simulink model "singleMassMPCDemodiscrete2017"  (R2017a)
settings: Solver=ode4  StartTime=0.0  StopTime=8  FixedStep=0.1  RelTol=1e-3
libraries: simulink x1
settings Model: Creator=daoist  LastModifiedBy=daoist
settings DataIOCC: ReturnWorkspaceOutputs=on
settings DebuggingCC: SFMachineParentedDataDiag=error
settings SFSimCC: SimUseLocalCustomCode=on
settings RTWCC: RTWUseLocalCustomCode=on

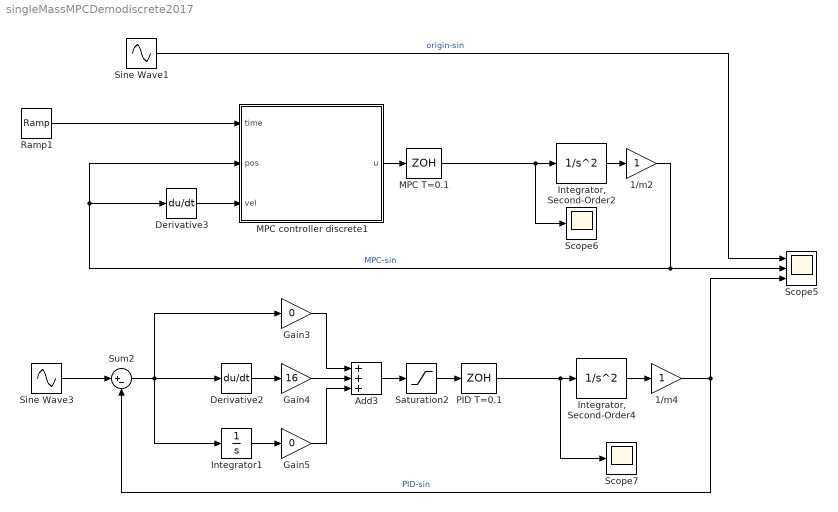
== system singleMassMPCDemodiscrete2017 ==
  1/m2 : Gain
  1/m4 : Gain
  Add3 : Sum  Inputs=+++
  Derivative2 : Derivative
  Derivative3 : Derivative
  Gain3 : Gain  Gain=0
  Gain4 : Gain  Gain=16
  Gain5 : Gain  Gain=0
  "Integrator, Second-Order2" : SecondOrderIntegrator  ShowOutput=x
  "Integrator, Second-Order4" : SecondOrderIntegrator  ShowOutput=x
  Integrator1 : Integrator
  MPC T=0.1 : ZeroOrderHold  SampleTime=0.1
  MPC controller discrete1 : MATLAB Function  TreatAsAtomicUnit=on
  PID T=0.1 : ZeroOrderHold  SampleTime=0.1
  Ramp1 : simulink/Sources/Ramp  slope=1  start=0  X0=0
  Saturation2 : Saturate  UpperLimit=100  LowerLimit=-100
  Scope5 : Scope  NumInputPorts=3
  Scope6 : Scope
  Scope7 : Scope
  Sine Wave1 : Sin  Frequency=pi  SampleTime=0
  Sine Wave3 : Sin  Frequency=pi  SampleTime=0
  Sum2 : Sum  Inputs=|+-
  wires:
  PID T=0.1/1 -> Scope7/1, "Integrator, Second-Order4"/1
  MPC T=0.1/1 -> Scope6/1, "Integrator, Second-Order2"/1
  Sum2/1 -> Derivative2/1, Integrator1/1, Gain3/1
  MPC controller discrete1/1(u) -> MPC T=0.1/1
  Gain4/1 -> Add3/2
  1/m4/1 -> Scope5/3, Sum2/2  "PID-sin"
  Sine Wave3/1 -> Sum2/1
  Gain5/1 -> Add3/3
  "Integrator, Second-Order4"/1 -> 1/m4/1
  Add3/1 -> Saturation2/1
  Saturation2/1 -> PID T=0.1/1
  Gain3/1 -> Add3/1
  Sine Wave1/1 -> Scope5/1  "origin-sin"
  Derivative2/1 -> Gain4/1
  Ramp1/1 -> MPC controller discrete1/1(time)
  Integrator1/1 -> Gain5/1
  "Integrator, Second-Order2"/1 -> 1/m2/1
  Derivative3/1 -> MPC controller discrete1/3(vel)
  1/m2/1 -> Scope5/2, Derivative3/1, MPC controller discrete1/2(pos)  "MPC-sin"

== matlab function singleMassMPCDemodiscrete2017/MPC controller discrete1 ==
  data: time input; pos input size=1; vel input size=1; u output size=1
function u = MPCcontrollerDiscrete( time, pos, vel)
%参数设置
m    = 1.05;          %滑块质量,增加了5%作为建模误差
T    = 0.1;           %控制周期100ms
p    = 40;            %控制时域（预测时域）
Q    = 10*eye(2*p);   %累计误差权重
W    = 0.0001*eye(p); %控制输出权重
% umax = 100;          
umax = 100 * ones(p,1); %控制量限制，即最大的力
Rk   = zeros(2*p,1);  %参考值序列
timeseris = time:T:time+T*(p-1);
Rk(1:2:end) = sin(pi()*(timeseris+T));    
Rk(2:2:end) = pi()*cos(pi()*(timeseris+T));    %参考速度
%构建中间变量
xk    = [pos;vel];    %xk
A_    = [1 T;0 1];    %离散化预测模型参数A
B_    = [0;T/m];      %离散化预测模型参数B
B_    = [T^2/m/2;T/m]; 
psi   = zeros(2*p,2); %psi
for i=1:1:p
    psi(i*2-1:i*2,1:2)=A_^i;
end
theta = zeros(2*p,p); %theta
for i=1:1:p
    for j=1:1:i
        theta(i*2-1:i*2,j)=A_^(i-j)*B_;
    end
end
E = psi*xk-Rk;            %E
H = 2*(theta'*Q*theta+W); %H
f = (2*E'*Q*theta)';      %f
%优化求解
coder.extrinsic('quadprog');
Uk=quadprog(H,f,[],[],[],[],-umax,umax);
%返回控制量序列第一个值
u = 0.0;                %显示指定u的类型
u = Uk(1);
